simulink model "GFM_GFL_referenceModel_mss_sfunc"  (R2023b)
settings: Solver=ode23  StartTime=0.1  StopTime=1  MaxStep=SimulationSetup.Solver.MaxStep  RelTol=SimulationSetup.Solver.RelTol
undefined symbols (not defined in the file): freq, H, Ibase, K_damping, Kdroop_V, Ki_CC, ki_P, ki_PLL, ki_Q, Kp_CC, kp_P, kp_PLL, kp_Q, Lconv1, Lg, Lv, msys, Qref, Rconv1, Rg, Rv, Sbase, SimulationSetup, Vpeak, wf_PQ, wg, x0
libraries: eeStairGenerator x1
settings Model: Creator=kauchr  LastModifiedBy=weq968
settings DataIOCC: ExternalInput=[tsig, usig]  LoadInitialState=on  SaveFinalState=on  SaveOperatingPoint=on  SaveState=on

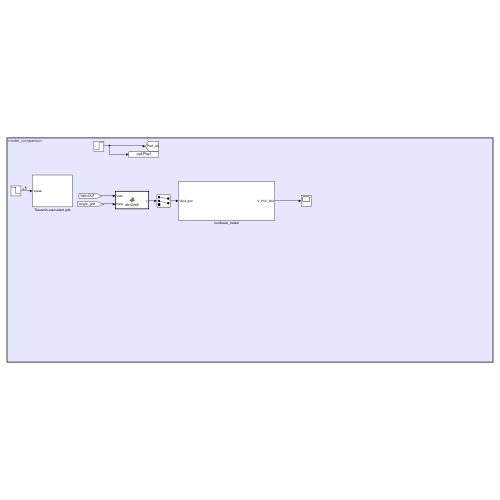
[thumbnail: Simulink's stored preview of the top-level diagram]
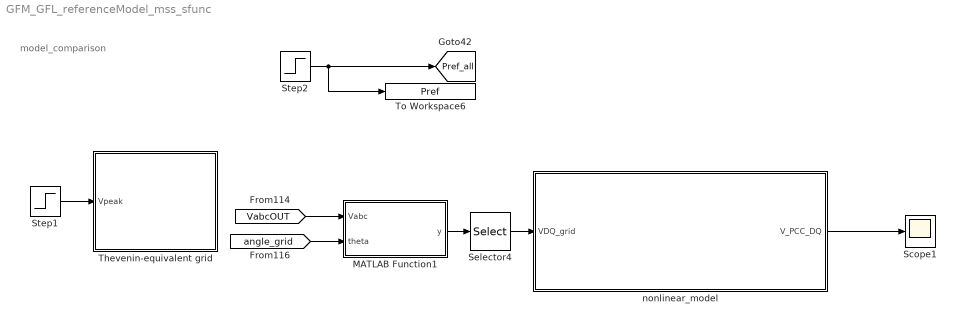
== system GFM_GFL_referenceModel_mss_sfunc ==
  note: model_comparison
  MATLAB Function1 : MATLAB Function  TreatAsAtomicUnit=on
  Scope1 : Scope
  Selector4 : Selector  InputPortWidth=3  IndexOptions=Index vector (dialog)  Indices=[1 2]  OutputSizes=1
  Step1 : Step  Time=SimulationSetup.grid.voltageAmplitudeStep.Time  Before=SimulationSetup.grid.voltageAmplitudeStep.Values(1)  After=SimulationSetup.grid.voltageAmplitudeStep.Values(2)  SampleTime=0
  Step2 : Step  Time=SimulationSetup.converter1.Pref.Time  Before=SimulationSetup.converter1.Pref.Values(1)  After=SimulationSetup.converter1.Pref.Values(2)  SampleTime=0
  Thevenin-equivalent grid : Subsystem
  To Workspace6 : ToWorkspace  VariableName=Pref  SaveFormat=Timeseries  SampleTime=-1
      settings: Save2DSignal=2-D array (concatenate along first dimension)
  nonlinear_model : Subsystem
  tag scope: Pref_all=global
  wires:
  nonlinear_model/1(V_PCC_DQ) -> Scope1/1
  Selector4/1 -> nonlinear_model/1(VDQ_grid)
  [VabcOUT] -> MATLAB Function1/1(Vabc)
  MATLAB Function1/1(y) -> Selector4/1
  [angle_grid] -> MATLAB Function1/2(theta)
  Step1/1 -> Thevenin-equivalent grid/1(Vpeak)
  Step2/1 -> To Workspace6/1, [Pref_all]

== system GFM_GFL_referenceModel_mss_sfunc/Thevenin-equivalent grid ==
  Vpeak : Inport
  Grid : Subsystem
  Mux : Mux  Inputs=3
  tag scope: VabcOUT=global, angle_grid=global
  wires:
  Grid/4(thetareal) -> [angle_grid]
  Grid/2(vzb) -> Mux/2
  Grid/3(vzc) -> Mux/3
  Mux/1 -> [VabcOUT]
  Grid/1(vza) -> Mux/1
  Vpeak/1 -> Grid/1(Vpeak)

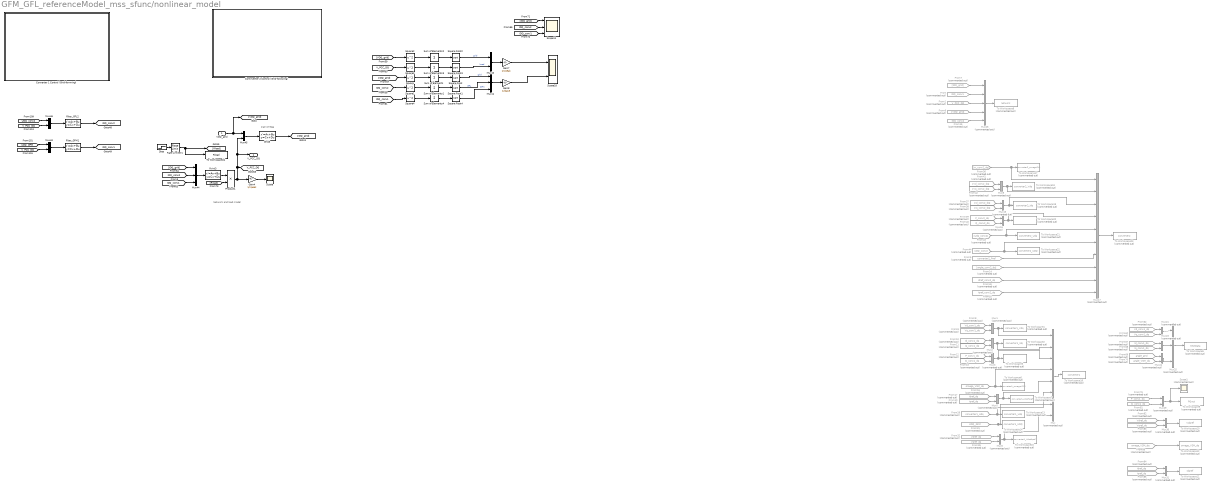
== system GFM_GFL_referenceModel_mss_sfunc/nonlinear_model ==
  note: Network and load model
  note: sign omega
  VDQ_grid : Inport
  Comnverter 2 Control (Grid-following) : Subsystem
  Converter 1 Control (Grid-forrming) : Subsystem
  From : From  Commented=on  GotoTag=IDQ_conv1  TagVisibility=global
  From1 : From  Commented=on  GotoTag=V_PCC_DQ  TagVisibility=global
  From10 : From  Commented=on  GotoTag=Id_conv1_dq  TagVisibility=global
  From11 : From  Commented=on  GotoTag=Iq_conv1_dq  TagVisibility=global
  From12 : From  Commented=on  GotoTag=P_conv1_dq  TagVisibility=global
  From13 : From  Commented=on  GotoTag=Q_conv1_dq  TagVisibility=global
  From14 : From  Commented=on  GotoTag=angle_conv2_dq  TagVisibility=global
  From15 : From  Commented=on  GotoTag=IDQ_conv2  TagVisibility=global
  From16 : From  Commented=on  GotoTag=omega_VSM_dq  TagVisibility=global
  From17 : From  Commented=on  GotoTag=Idref_dq  TagVisibility=global
  From18 : From  Commented=on  GotoTag=Iqref_dq  TagVisibility=global
  From26 : From  Commented=on  GotoTag=converter1_Udq  TagVisibility=global
  From31 : From  Commented=on  GotoTag=UDQ_GFM  TagVisibility=global
  From32 : From  Commented=on  GotoTag=Vdref_dq  TagVisibility=global
  From35 : From  Commented=on  GotoTag=Vqref_dq  TagVisibility=global
  From36 : From  Commented=on  GotoTag=w_conv2_dq  TagVisibility=global
  From37 : From  Commented=on  GotoTag=Id_conv2_dq  TagVisibility=global
  From38 : From  Commented=on  GotoTag=Iq_conv2_dq  TagVisibility=global
  From39 : From  Commented=on  GotoTag=P_conv2_dq  TagVisibility=global
  From40 : From  Commented=on  GotoTag=Q_conv2_dq  TagVisibility=global
  From41 : From  Commented=on  GotoTag=Vd_conv2_dq
  From42 : From  Commented=on  GotoTag=Vq_conv2_dq
  From43 : From  Commented=on  GotoTag=Udq_conv2  TagVisibility=global
  From44 : From  Commented=on  GotoTag=UDQ_conv2  TagVisibility=global
  From45 : From  Commented=on  GotoTag=Idref_conv2_dq  TagVisibility=global
  From5 : From  Commented=on  GotoTag=converter2_Pref  TagVisibility=global
  From55 : From  Commented=on  GotoTag=Iqref_conv2_dq  TagVisibility=global
  From6 : From  Commented=on  GotoTag=VDQ_grid
  From62 : From  Commented=on  GotoTag=Vd_conv1_dq  TagVisibility=global
  From63 : From  Commented=on  GotoTag=Vq_conv1_dq  TagVisibility=global
  From67 : From  Commented=on  GotoTag=Id_conv1_dq  TagVisibility=global
  From68 : From  Commented=on  GotoTag=Iq_conv1_dq  TagVisibility=global
  From69 : From  Commented=on  GotoTag=angle_grid  TagVisibility=global
  From7 : From  Commented=on  GotoTag=IDQ_grid
  From70 : From  Commented=on  GotoTag=angle_VSM_dq  TagVisibility=global
  From76 : From  Commented=on  GotoTag=P_conv1_dq  TagVisibility=global
  From8 : From  Commented=on  GotoTag=Vd_conv1_dq  TagVisibility=global
  From81 : From  Commented=on  GotoTag=Q_conv1_dq  TagVisibility=global
  From82 : From  Commented=on  GotoTag=Vdref_dq  TagVisibility=global
  From83 : From  Commented=on  GotoTag=Vqref_dq  TagVisibility=global
  From84 : From  Commented=on  GotoTag=Idref_dq  TagVisibility=global
  From85 : From  Commented=on  GotoTag=Iqref_dq  TagVisibility=global
  From88 : From  Commented=on  GotoTag=omega_VSM_dq  TagVisibility=global
  From9 : From  Commented=on  GotoTag=Vq_conv1_dq  TagVisibility=global
  Gain4 : Gain  Gain=1/Vpeak
  Gain7 : Gain  Gain=1/Vpeak
  Gain8 : Gain  Gain=1/Ibase
  Grid3 : StateSpace  A=[-Rg/Lg wg; -wg -Rg/Lg]  B=1/Lg*[eye(2),-eye(2)]  C=eye(2)  D=zeros(2,4)  InitialCondition=0  ContinuousStateAttributes='grid_IDQ'
  Mux : Mux  Commented=on  Inputs=[2 2 2 1 2 2 2 2]
  Mux{1..3,5..6,9,15..16,21,23..24,29..31} (14 alike) : Mux  Commented=on  Inputs=2
  Mux10 : Mux  Inputs=2
  Mux11 : Mux  Inputs=3
  Mux17 : Mux  Commented=on  Inputs=[1 2 2 2 2 2 1 1 1 1]
  Mux25 : Mux  Commented=on  Inputs=3
  Mux26 : Mux  Commented=on  Inputs=5
  Mux43 : Mux  Inputs=[2 2]
  Mux44 : Mux  Inputs=[2 2 2]
  Mux45 : Mux  Inputs=[2 2]
  Mux46 : Mux  Inputs=[2 2]
  Product1 : Product
  Rate Limiter1 : RateLimiter  RisingSlewLimit=1000000  FallingSlewLimit=-1000000  SampleTimeMode=inherited
  Rvirt3 : StateSpace  A=[]  B=[]  C=[]  D=[eye(2),eye(2),eye(2)]  InitialCondition=0  ContinuousStateAttributes='VDQ_PCC'
  Scope : Scope
  Scope1 : Scope  Commented=on
  Scope11 : Scope  NumInputPorts=3
  Scope18 : Scope  NumInputPorts=2
  Square{,1..4} (5 alike) : Math  Operator=square
  Square Root{,1..4} (5 alike) : Sqrt
  Step : Step  Time=SimulationSetup.Load.Step.Time  Before=SimulationSetup.Load.Base  After=SimulationSetup.Load.Step.Value  SampleTime=0
  Sum of Elements{,1..4} (5 alike) : Sum  Inputs=+
  To Workspace1 : ToWorkspace  Commented=on  VariableName=converter1_Vdq  SaveFormat=Structure With Time  SampleTime=-1
  To Workspace10 : ToWorkspace  Commented=on  VariableName=Vdqref  SaveFormat=Timeseries  SampleTime=-1
      settings: Save2DSignal=2-D array (concatenate along first dimension)
  To Workspace11 : ToWorkspace  Commented=on  VariableName=Idqref  SaveFormat=Timeseries  SampleTime=-1
      settings: Save2DSignal=2-D array (concatenate along first dimension)
  To Workspace12 : ToWorkspace  Commented=on  VariableName=omega_VSM_dq  SaveFormat=Timeseries  SampleTime=-1
      settings: Save2DSignal=2-D array (concatenate along first dimension)
  To Workspace13 : ToWorkspace  Commented=on  VariableName=converter1_Udq  SaveFormat=Timeseries  SampleTime=-1
      settings: Save2DSignal=2-D array (concatenate along first dimension)
  To Workspace14 : ToWorkspace  Commented=on  VariableName=converter1_UDQ  SaveFormat=Timeseries  SampleTime=-1
      settings: Save2DSignal=2-D array (concatenate along first dimension)
  To Workspace15 : ToWorkspace  Commented=on  VariableName=converter1_Vdrefqref  SaveFormat=Timeseries  SampleTime=-1
      settings: Save2DSignal=2-D array (concatenate along first dimension)
  To Workspace16 : ToWorkspace  Commented=on  VariableName=converter1  SaveFormat=Structure With Time  SampleTime=-1
  To Workspace17 : ToWorkspace  Commented=on  VariableName=converter2_omegaPLL  SaveFormat=Timeseries  SampleTime=-1
      settings: Save2DSignal=2-D array (concatenate along first dimension)
  To Workspace18 : ToWorkspace  Commented=on  VariableName=converter2_Vdq  SaveFormat=Structure With Time  SampleTime=-1
  To Workspace19 : ToWorkspace  Commented=on  VariableName=converter2_Idq  SaveFormat=Structure With Time  SampleTime=-1
  To Workspace2 : ToWorkspace  Commented=on  VariableName=converter1_Idq  SaveFormat=Structure With Time  SampleTime=-1
  To Workspace20 : ToWorkspace  Commented=on  VariableName=converter2_PmeasQmeas  SaveFormat=Structure With Time  SampleTime=-1
  To Workspace21 : ToWorkspace  Commented=on  VariableName=converter2_Udq  SaveFormat=Timeseries  SampleTime=-1
      settings: Save2DSignal=2-D array (concatenate along first dimension)
  To Workspace22 : ToWorkspace  Commented=on  VariableName=converter2_UDQ  SaveFormat=Timeseries  SampleTime=-1
      settings: Save2DSignal=2-D array (concatenate along first dimension)
  To Workspace23 : ToWorkspace  Commented=on  VariableName=converter2  SaveFormat=Structure  SampleTime=-1
      settings: Save2DSignal=2-D array (concatenate along first dimension)
  To Workspace24 : ToWorkspace  VariableName=Rload  SaveFormat=Timeseries  SampleTime=-1
      settings: Save2DSignal=2-D array (concatenate along first dimension)
  To Workspace3 : ToWorkspace  Commented=on  VariableName=converter1_PmeasQmeas  SaveFormat=Structure With Time  SampleTime=-1
  To Workspace5 : ToWorkspace  Commented=on  VariableName=testData  SaveFormat=Structure With Time  SampleTime=-1
  To Workspace6 : ToWorkspace  Commented=on  VariableName=converter1_omegaVSM  SaveFormat=Timeseries  SampleTime=-1
      settings: Save2DSignal=2-D array (concatenate along first dimension)
  To Workspace7 : ToWorkspace  Commented=on  VariableName=converter1_IdrefIqref  SaveFormat=Timeseries  SampleTime=-1
      settings: Save2DSignal=2-D array (concatenate along first dimension)
  To Workspace8 : ToWorkspace  Commented=on  VariableName=network  SaveFormat=Timeseries  SampleTime=-1
      settings: Save2DSignal=2-D array (concatenate along first dimension)
  To Workspace9 : ToWorkspace  Commented=on  VariableName=PQout  SaveFormat=Timeseries  SampleTime=-1
      settings: Save2DSignal=2-D array (concatenate along first dimension)
  filter_GFL2 : StateSpace  A=[-Rconv1/Lconv1 wg; -wg -Rconv1/Lconv1]  B=1/Lconv1*[eye(2),-eye(2)]  C=eye(2)  D=zeros(2,4)  InitialCondition=0  ContinuousStateAttributes='converter2_IDQ'
  filter_GFM1 : StateSpace  A=[-Rconv1/Lconv1 wg; -wg -Rconv1/Lconv1]  B=1/Lconv1*[eye(2),-eye(2)]  C=eye(2)  D=zeros(2,4)  InitialCondition=0  ContinuousStateAttributes='converter1_IDQ'
  V_PCC_DQ : Outport
  tag scope: IDQ_conv1=global, IDQ_conv2=global, V_PCC_DQ=global
  wires:
  Mux29/1 -> Scope1/1, To Workspace9/1
  Mux30/1 -> To Workspace10/1
  Mux31/1 -> To Workspace11/1
  From81/1 -> Mux29/2
  From85/1 -> Mux31/2
  From82/1 -> Mux30/1
  From88/1 -> To Workspace12/1
  From84/1 -> Mux31/1
  From83/1 -> Mux30/2
  From76/1 -> Mux29/1
  From36/1 -> Mux17/1, To Workspace17/1
  From41/1 -> Mux9/1
  Mux9/1 -> Mux17/2, To Workspace18/1
  Mux15/1 -> Mux17/3, To Workspace19/1
  From39/1 -> Mux16/1
  From42/1 -> Mux9/2
  Mux16/1 -> Mux17/4, To Workspace20/1
  From40/1 -> Mux16/2
  From38/1 -> Mux15/2
  From37/1 -> Mux15/1
  From43/1 -> Mux17/5, To Workspace21/1
  From44/1 -> Mux17/6, To Workspace22/1
  Mux17/1 -> To Workspace23/1
  From5/1 -> Mux17/7
  From14/1 -> Mux17/8
  From45/1 -> Mux17/9
  From55/1 -> Mux17/10
  Step/1 -> Rate Limiter1/1
  Gain4/1 -> Scope/1
  filter_GFL2/1 -> [IDQ_conv2]
  [UDQ_conv2] -> Mux46/1
  Mux45/1 -> Grid3/1
  Rvirt3/1 -> Product1/1
  [V_PCC_DQ] -> Mux43/2
  VDQ_grid/1 -> Mux45/1, [VDQ_grid]
  Rate Limiter1/1 -> To Workspace24/1, [Rload]
  Mux43/1 -> filter_GFM1/1
  Grid3/1 -> [IDQ_grid]
  Mux46/1 -> filter_GFL2/1
  [IDQ_conv1] -> Mux44/3
  Product1/1 -> Gain4/1, Mux45/2, V_PCC_DQ/1, [V_PCC_DQ]
  Mux44/1 -> Rvirt3/1
  [UDQ_GFM] -> Mux43/1
  [V_PCC_DQ] -> Mux46/2
  [IDQ_conv2] -> Mux44/2
  [IDQ_grid] -> Mux44/1
  filter_GFM1/1 -> [IDQ_conv1]
  [Rload] -> Product1/2
  Mux5/1 -> Mux/5, To Workspace7/1
  From18/1 -> Mux5/2
  From11/1 -> Mux2/2
  Mux2/1 -> Mux/2, To Workspace2/1
  From13/1 -> Mux3/2
  Mux1/1 -> Mux/1, To Workspace1/1
  Mux3/1 -> Mux/3, To Workspace3/1
  From32/1 -> Mux6/1
  From12/1 -> Mux3/1
  From26/1 -> Mux/6, To Workspace13/1
  Mux6/1 -> Mux/8, To Workspace15/1
  From17/1 -> Mux5/1
  From16/1 -> Mux/4, To Workspace6/1
  From8/1 -> Mux1/1
  From35/1 -> Mux6/2
  From10/1 -> Mux2/1
  Mux/1 -> To Workspace16/1
  From9/1 -> Mux1/2
  From31/1 -> Mux/7, To Workspace14/1
  From62/1 -> Mux21/1
  From70/1 -> Mux24/2
  From68/1 -> Mux23/2
  Mux24/1 -> Mux25/3
  From69/1 -> Mux24/1
  From67/1 -> Mux23/1
  Mux21/1 -> Mux25/1
  Mux23/1 -> Mux25/2
  Mux25/1 -> To Workspace5/1
  From63/1 -> Mux21/2
  From15/1 -> Mux26/5
  Mux26/1 -> To Workspace8/1
  From1/1 -> Mux26/3
  From/1 -> Mux26/2
  From6/1 -> Mux26/4
  From7/1 -> Mux26/1
  [IDQ_grid] -> Scope11/1
  [IDQ_conv1] -> Scope11/3
  [IDQ_conv2] -> Scope11/2
  [IDQ_grid] -> Square/1
  Gain7/1 -> Scope18/1
  [V_PCC_DQ] -> Square3/1
  Mux11/1 -> Gain8/1
  [IDQ_conv1] -> Square4/1
  Sum of Elements1/1 -> Square Root1/1
  Square Root4/1 -> Mux11/3  "GFM"
  Square Root2/1 -> Mux10/1  "grid"
  [VDQ_grid] -> Square2/1
  Square2/1 -> Sum of Elements2/1
  Square/1 -> Sum of Elements/1
  Square Root1/1 -> Mux11/2  "GFL"
  Square1/1 -> Sum of Elements1/1
  Square Root3/1 -> Mux10/2  "load"
  Sum of Elements/1 -> Square Root/1
  Gain8/1 -> Scope18/2
  Mux10/1 -> Gain7/1
  [IDQ_conv2] -> Square1/1
  Sum of Elements3/1 -> Square Root3/1
  Square Root/1 -> Mux11/1  "grid"
  Sum of Elements2/1 -> Square Root2/1
  Sum of Elements4/1 -> Square Root4/1
  Square3/1 -> Sum of Elements3/1
  Square4/1 -> Sum of Elements4/1

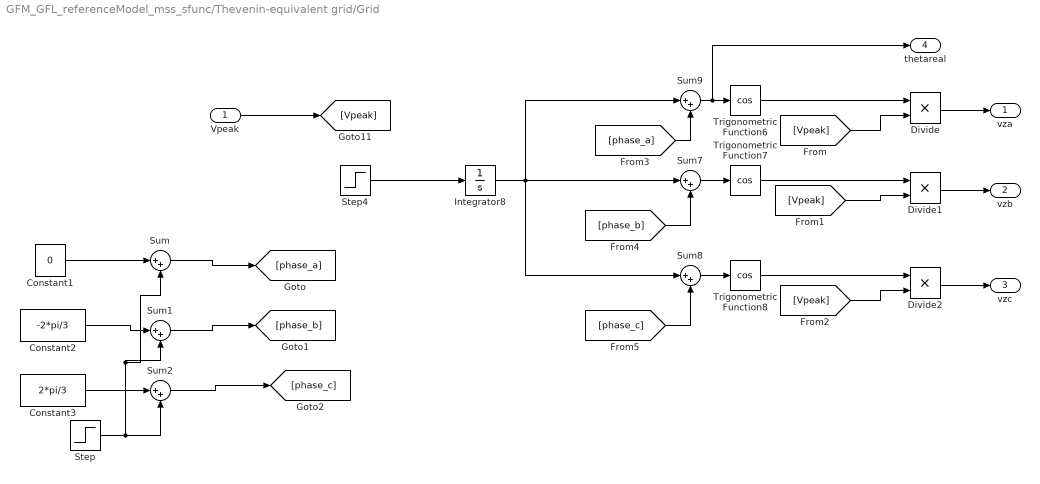
== system GFM_GFL_referenceModel_mss_sfunc/Thevenin-equivalent grid/Grid ==
  Vpeak : Inport
  Constant1 : Constant  Value=0
  Constant2 : Constant  Value=-2*pi/3
  Constant3 : Constant  Value=2*pi/3
  Divide : Product  Inputs=**
  Divide1 : Product  Inputs=**
  Divide2 : Product  Inputs=**
  Integrator8 : Integrator  ContinuousStateAttributes='grid_thetaGRID'
  Step : Step  Time=SimulationSetup.grid.PhaseStep.Time  Before=SimulationSetup.grid.PhaseStep.Values(1)  After=SimulationSetup.grid.PhaseStep.Values(2)  SampleTime=0
  Step4 : Step  Time=SimulationSetup.grid.FrequencyStep.Time  Before=SimulationSetup.grid.FrequencyStep.Values(1)  After=SimulationSetup.grid.FrequencyStep.Values(2)  SampleTime=0
  Sum{,1..2,7..9} (6 alike) : Sum  Inputs=|++
  Trigonometric Function6 : Trigonometry  Operator=cos
  Trigonometric Function7 : Trigonometry  Operator=cos
  Trigonometric Function8 : Trigonometry  Operator=cos
  vza : Outport
  vzb : Outport  Port=2
  vzc : Outport  Port=3
  thetareal : Outport  Port=4
  wires:
  Sum9/1 -> thetareal/1, Trigonometric Function6/1
  [phase_c] -> Sum8/2
  Integrator8/1 -> Sum8/1, Sum9/1, Sum7/1
  [phase_b] -> Sum7/2
  Sum7/1 -> Trigonometric Function7/1
  [phase_a] -> Sum9/2
  Sum8/1 -> Trigonometric Function8/1
  Trigonometric Function6/1 -> Divide/1
  Trigonometric Function7/1 -> Divide1/1
  Trigonometric Function8/1 -> Divide2/1
  Divide/1 -> vza/1
  Divide1/1 -> vzb/1
  Divide2/1 -> vzc/1
  [Vpeak] -> Divide/2
  [Vpeak] -> Divide1/2
  [Vpeak] -> Divide2/2
  Sum1/1 -> [phase_b]
  Sum/1 -> [phase_a]
  Constant1/1 -> Sum/1
  Constant2/1 -> Sum1/1
  Constant3/1 -> Sum2/1
  Sum2/1 -> [phase_c]
  Step/1 -> Sum/2, Sum1/2, Sum2/2
  Step4/1 -> Integrator8/1
  Vpeak/1 -> [Vpeak]

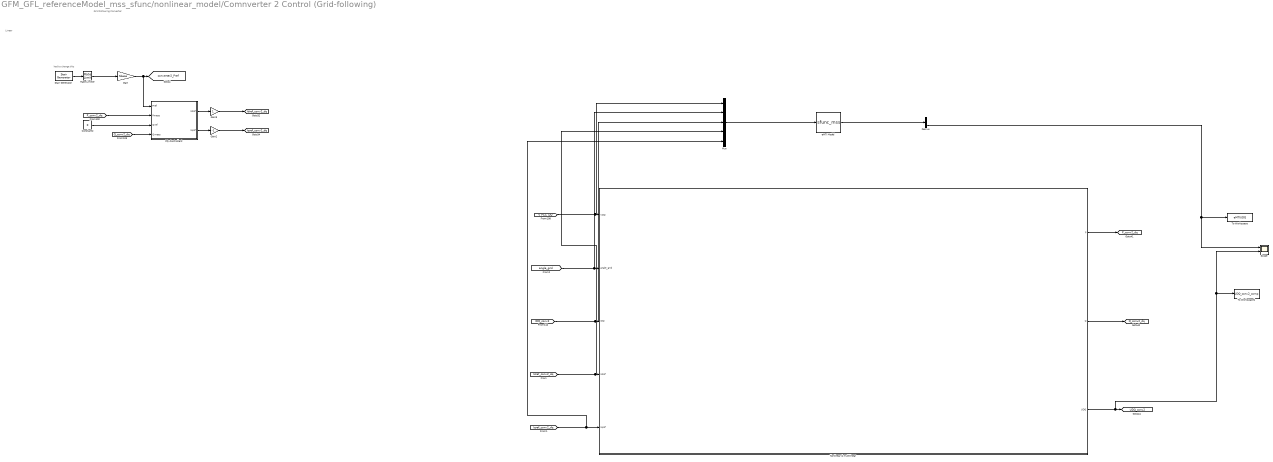
== system GFM_GFL_referenceModel_mss_sfunc/nonlinear_model/Comnverter 2 Control (Grid-following) ==
  note: Linear
  note: Grid Following Converter
  note: had to change this
  Constant2 : Constant  Value=0
  Demux : Demux  Outputs=[1 1 2]
  Gain : Gain  Gain=Sbase
  Gain2 : Gain  Gain=-1
  Gain3 : Gain
  Mux : Mux  Inputs=[2 1 2 1 1]
  Nonlinear & multilinear : Subsystem
  PQ-Controller2 : Subsystem
  Rate Limiter : RateLimiter  RisingSlewLimit=100  FallingSlewLimit=-100  SampleTimeMode=inherited
  Scope : Scope  NumInputPorts=2
  Stair Generator : eeStairGenerator/Stair Generator  LabelModeActiveChoice=Continuous  TimeInput=SimulationSetup.converter2.Pref.Time  AmplitudeInput=SimulationSetup.converter2.Pref.Values  SampleTime=0  RepeatPattern=off  OutDataTypeStr=double
      settings: LibrarySourceBlock=ee_sl_lib/General Control/Stair Generator
  To Workspace : ToWorkspace  VariableName=eMTIUDQ  SaveFormat=Timeseries  SampleTime=-1
  To Workspace1 : ToWorkspace  VariableName=UDQ_conv2_comp  SaveFormat=Timeseries  SampleTime=-1
  eMTI Model : M-S-Function  FunctionName=sfunc_mss  Parameters=msys,x0  mask{msys=msys, x0=x0}
      mask prompts: msys "eMTI model"; x0 "Initial state"
      mask DialogControl eMTI Prompt: This is an implementation of an explicit multilinear (eMTI) model
      mask Display:
      | text(0.5,0.5,'eMTI',...
      |     horizontalAlignment='cente', ...
      |     verticalAlignment = 'middle')
  tag scope: Idref_conv2_dq=global, Iqref_conv2_dq=global, P_conv2_dq=global, Q_conv2_dq=global, UDQ_conv2=global, converter2_Pref=global
  wires:
  PQ-Controller2/2(Iqref) -> Gain2/1
  Gain2/1 -> [Iqref_conv2_dq]
  Gain/1 -> [converter2_Pref], PQ-Controller2/1(Pref)
  Gain3/1 -> [Idref_conv2_dq]
  [P_conv2_dq] -> PQ-Controller2/2(Pmeas)
  PQ-Controller2/1(Idref) -> Gain3/1
  [Q_conv2_dq] -> PQ-Controller2/4(Qmeas)
  Rate Limiter/1 -> Gain/1
  Constant2/1 -> PQ-Controller2/3(Qref)
  Stair Generator/1 -> Rate Limiter/1
  Nonlinear & multilinear/1(P) -> [P_conv2_dq]
  Nonlinear & multilinear/2(Q) -> [Q_conv2_dq]
  [V_PCC_DQ] -> Mux/1, Nonlinear & multilinear/1(VDQ)
  [angle_grid] -> Mux/2, Nonlinear & multilinear/2(angle_grid)
  [IDQ_conv2] -> Mux/3, Nonlinear & multilinear/3(IDQ)
  [Iqref_conv2_dq] -> Mux/5, Nonlinear & multilinear/5(Iqref)
  Nonlinear & multilinear/3(UDQ) -> To Workspace1/1, Scope/2, [UDQ_conv2]
  [Idref_conv2_dq] -> Mux/4, Nonlinear & multilinear/4(Idref)
  Mux/1 -> eMTI Model/1
  eMTI Model/1 -> Demux/1
  Demux/3 -> Scope/1, To Workspace/1

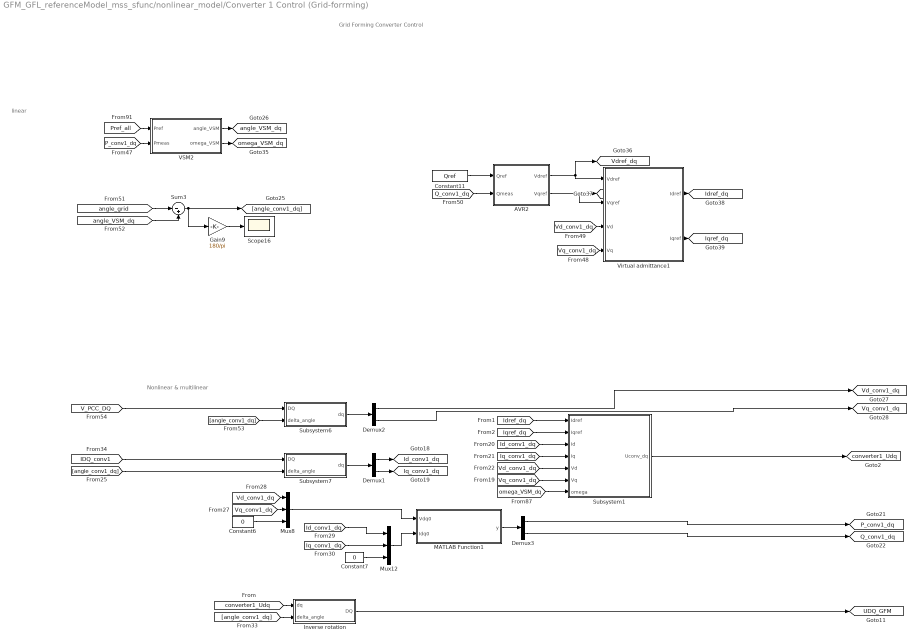
== system GFM_GFL_referenceModel_mss_sfunc/nonlinear_model/Converter 1 Control (Grid-forrming) ==
  note: linear
  note: Nonlinear & multilinear
  note: Grid Forming Converter Control
  AVR2 : Subsystem
  Constant11 : Constant  Value=Qref
  Constant6 : Constant  Value=0
  Constant7 : Constant  Value=0
  Demux1 : Demux  Outputs=2
  Demux2 : Demux  Outputs=2
  Demux3 : Demux  Outputs=2
  Gain9 : Gain  Gain=180/pi
  Inverse rotation : Subsystem
  MATLAB Function1 : MATLAB Function  TreatAsAtomicUnit=on
  Mux12 : Mux  Inputs=3
  Mux8 : Mux  Inputs=3
  Scope16 : Scope
  Subsystem1 : Subsystem
  Subsystem6 : Subsystem
  Subsystem7 : Subsystem
  Sum3 : Sum  Inputs=|-+
  VSM2 : Subsystem
  Virtual admittance1 : Subsystem
  tag scope: Id_conv1_dq=global, Idref_dq=global, Iq_conv1_dq=global, Iqref_dq=global, P_conv1_dq=global, Q_conv1_dq=global, UDQ_GFM=global, Vd_conv1_dq=global, Vdref_dq=global, Vq_conv1_dq=global, Vqref_dq=global, angle_VSM_dq=global, converter1_Udq=global, omega_VSM_dq=global
  wires:
  Virtual admittance1/2(Iqref) -> [Iqref_dq]
  [angle_conv1_dq] -> Inverse rotation/2(delta_angle)
  [Id_conv1_dq] -> Subsystem1/3(Id)
  Mux12/1 -> MATLAB Function1/2(Idq0)
  Sum3/1 -> Gain9/1, [angle_conv1_dq]
  Constant6/1 -> Mux8/3
  Constant11/1 -> AVR2/1(Qref)
  [Id_conv1_dq] -> Mux12/1
  [IDQ_conv1] -> Subsystem7/1(DQ)
  [Vq_conv1_dq] -> Subsystem1/6(Vq)
  [V_PCC_DQ] -> Subsystem6/1(DQ)
  [Vd_conv1_dq] -> Mux8/1
  [angle_conv1_dq] -> Subsystem7/2(delta_angle)
  AVR2/2(Vqref) -> [Vqref_dq], Virtual admittance1/2(Vqref)
  Subsystem1/1(Uconv_dq) -> [converter1_Udq]
  Mux8/1 -> MATLAB Function1/1(Vdq0)
  Gain9/1 -> Scope16/1
  AVR2/1(Vdref) -> [Vdref_dq], Virtual admittance1/1(Vdref)
  Demux1/1 -> [Id_conv1_dq]
  Virtual admittance1/1(Idref) -> [Idref_dq]
  VSM2/1(angle_VSM) -> [angle_VSM_dq]
  [Vd_conv1_dq] -> Virtual admittance1/3(Vd)
  VSM2/2(omega_VSM) -> [omega_VSM_dq]
  [angle_grid] -> Sum3/1
  [Vq_conv1_dq] -> Virtual admittance1/4(Vq)
  Constant7/1 -> Mux12/3
  Subsystem7/1(dq) -> Demux1/1
  [Iq_conv1_dq] -> Subsystem1/4(Iq)
  [P_conv1_dq] -> VSM2/2(Pmeas)
  [angle_conv1_dq] -> Subsystem6/2(delta_angle)
  Demux3/2 -> [Q_conv1_dq]
  [angle_VSM_dq] -> Sum3/2
  Inverse rotation/1(DQ) -> [UDQ_GFM]
  [Q_conv1_dq] -> AVR2/2(Qmeas)
  [Vq_conv1_dq] -> Mux8/2
  Subsystem6/1(dq) -> Demux2/1
  Demux2/2 -> [Vq_conv1_dq]
  Demux2/1 -> [Vd_conv1_dq]
  [Iq_conv1_dq] -> Mux12/2
  Demux1/2 -> [Iq_conv1_dq]
  [omega_VSM_dq] -> Subsystem1/7(omega)
  [Pref_all] -> VSM2/1(Pref)
  [Vd_conv1_dq] -> Subsystem1/5(Vd)
  [converter1_Udq] -> Inverse rotation/1(dq)
  [Idref_dq] -> Subsystem1/1(Idref)
  [Iqref_dq] -> Subsystem1/2(Iqref)
  MATLAB Function1/1(y) -> Demux3/1
  Demux3/1 -> [P_conv1_dq]

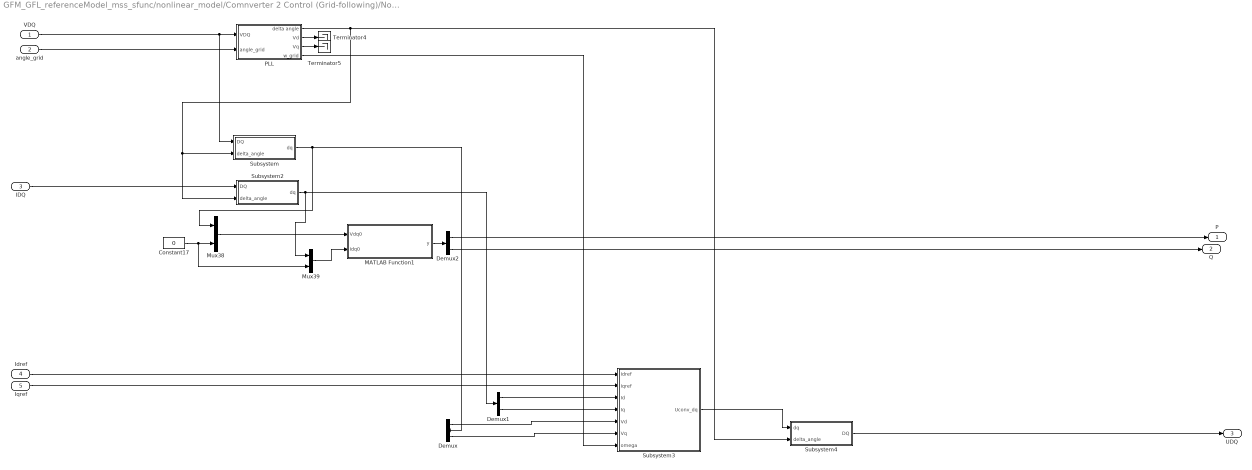
== system GFM_GFL_referenceModel_mss_sfunc/nonlinear_model/Comnverter 2 Control (Grid-following)/Nonlinear & multilinear ==
  VDQ : Inport
  angle_grid : Inport  Port=2
  IDQ : Inport  Port=3
  Idref : Inport  Port=4
  Iqref : Inport  Port=5
  Constant17 : Constant  Value=0
  Demux : Demux  Outputs=2
  Demux1 : Demux  Outputs=2
  Demux2 : Demux  Outputs=2
  MATLAB Function1 : MATLAB Function  TreatAsAtomicUnit=on
  Mux38 : Mux  Inputs=[2 1]
  Mux39 : Mux  Inputs=[2 1]
  PLL : Subsystem
  Subsystem : Subsystem
  Subsystem2 : Subsystem
  Subsystem3 : Subsystem
  Subsystem4 : Subsystem
  Terminator4 : Terminator
  Terminator5 : Terminator
  P : Outport
  Q : Outport  Port=2
  UDQ : Outport  Port=3
  wires:
  Iqref/1 -> Subsystem3/2(Iqref)
  PLL/1(delta angle) -> Subsystem2/2(delta_angle), Subsystem/2(delta_angle), Subsystem4/2(delta_angle)
  Subsystem/1(dq) -> Mux38/1, Demux/1
  Demux2/2 -> Q/1
  Subsystem4/1(DQ) -> UDQ/1
  Constant17/1 -> Mux39/2, Mux38/2
  Demux1/2 -> Subsystem3/4(Iq)
  VDQ/1 -> Subsystem/1(DQ), PLL/1(VDQ)
  Demux/2 -> Subsystem3/6(Vq)
  Subsystem2/1(dq) -> Mux39/1, Demux1/1
  PLL/4(w_grid) -> Subsystem3/7(omega)
  PLL/3(Vq) -> Terminator5/1
  PLL/2(Vd) -> Terminator4/1
  Idref/1 -> Subsystem3/1(Idref)
  Mux38/1 -> MATLAB Function1/1(Vdq0)
  Mux39/1 -> MATLAB Function1/2(Idq0)
  Subsystem3/1(Uconv_dq) -> Subsystem4/1(dq)
  Demux1/1 -> Subsystem3/3(Id)
  Demux/1 -> Subsystem3/5(Vd)
  Demux2/1 -> P/1
  IDQ/1 -> Subsystem2/1(DQ)
  angle_grid/1 -> PLL/2(angle_grid)
  MATLAB Function1/1(y) -> Demux2/1

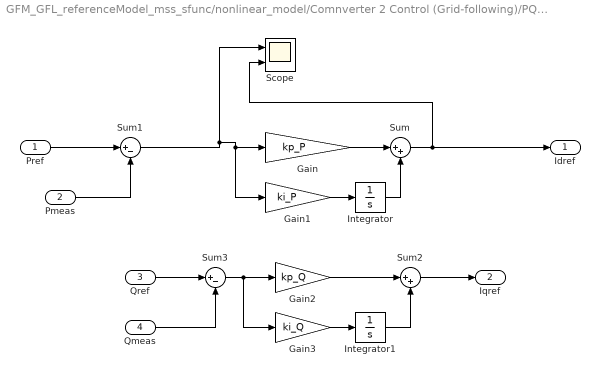
== system GFM_GFL_referenceModel_mss_sfunc/nonlinear_model/Comnverter 2 Control (Grid-following)/PQ-Controller2 ==
  Pref : Inport
  Pmeas : Inport  Port=2
  Qref : Inport  Port=3
  Qmeas : Inport  Port=4
  Gain : Gain  Gain=kp_P
  Gain1 : Gain  Gain=ki_P
  Gain2 : Gain  Gain=kp_Q
  Gain3 : Gain  Gain=ki_Q
  Integrator : Integrator  ContinuousStateAttributes='converter2_xI_Pctrl'
  Integrator1 : Integrator  ContinuousStateAttributes='converter2_xI_Qctrl'
  Scope : Scope  NumInputPorts=2
  Sum : Sum  Inputs=|++
  Sum1 : Sum  Inputs=|+-
  Sum2 : Sum  Inputs=|++
  Sum3 : Sum  Inputs=|+-
  Idref : Outport
  Iqref : Outport  Port=2
  wires:
  Gain1/1 -> Integrator/1
  Integrator/1 -> Sum/2
  Gain/1 -> Sum/1
  Sum/1 -> Idref/1, Scope/2
  Pmeas/1 -> Sum1/2
  Integrator1/1 -> Sum2/2
  Sum2/1 -> Iqref/1
  Sum3/1 -> Gain3/1, Gain2/1
  Gain2/1 -> Sum2/1
  Qmeas/1 -> Sum3/2
  Gain3/1 -> Integrator1/1
  Qref/1 -> Sum3/1
  Sum1/1 -> Scope/1, Gain1/1, Gain/1
  Pref/1 -> Sum1/1

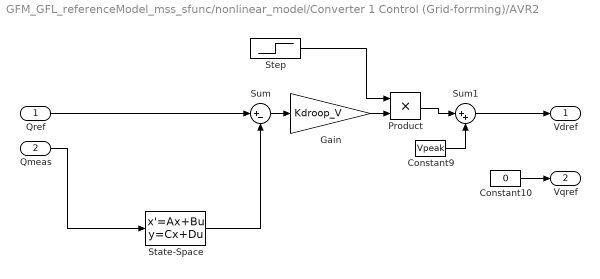
== system GFM_GFL_referenceModel_mss_sfunc/nonlinear_model/Converter 1 Control (Grid-forrming)/AVR2 ==
  Qref : Inport
  Qmeas : Inport  Port=2
  Constant10 : Constant  Value=0
  Constant9 : Constant  Value=Vpeak
  Gain : Gain  Gain=Kdroop_V
  Product : Product
  State-Space : StateSpace  A=-wf_PQ  B=wf_PQ  D=0  InitialCondition=0  ContinuousStateAttributes='converter1_xI_Vdroop'
  Step : Step  Time=SimulationSetup.converter1.VoltageCtrl.ActivationTime  SampleTime=0
  Sum : Sum  Inputs=|+-
  Sum1 : Sum  Inputs=|++
  Vdref : Outport
  Vqref : Outport  Port=2
  wires:
  Qref/1 -> Sum/1
  Constant9/1 -> Sum1/2
  Sum/1 -> Gain/1
  Qmeas/1 -> State-Space/1
  Product/1 -> Sum1/1
  Step/1 -> Product/1
  Gain/1 -> Product/2
  State-Space/1 -> Sum/2
  Sum1/1 -> Vdref/1
  Constant10/1 -> Vqref/1

== system GFM_GFL_referenceModel_mss_sfunc/nonlinear_model/Converter 1 Control (Grid-forrming)/Inverse rotation ==
  dq : Inport
  delta_angle : Inport  Port=2
  Gain : Gain
  Gain1 : Gain  Gain=-1
  Matrix Concatenate : Concatenate  Mode=Multidimensional array  ConcatenateDimension=2
  Mux : Mux  Inputs=2
  Mux1 : Mux  Inputs=2
  Product : Product  Multiplication=Matrix(*)
  Sin : Trigonometry
  Sin1 : Trigonometry  Operator=cos
  DQ : Outport
  wires:
  Matrix Concatenate/1 -> Product/1
  dq/1 -> Product/2
  Product/1 -> DQ/1
  delta_angle/1 -> Sin1/1, Sin/1
  Sin1/1 -> Mux1/2, Mux/1
  Sin/1 -> Gain1/1, Gain/1
  Gain/1 -> Mux/2
  Mux/1 -> Matrix Concatenate/1
  Mux1/1 -> Matrix Concatenate/2
  Gain1/1 -> Mux1/1

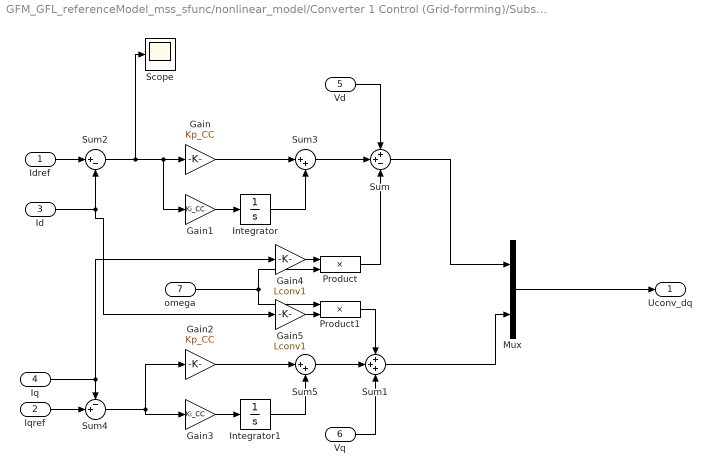
== system GFM_GFL_referenceModel_mss_sfunc/nonlinear_model/Converter 1 Control (Grid-forrming)/Subsystem1 ==
  Idref : Inport
  Iqref : Inport  Port=2
  Id : Inport  Port=3
  Iq : Inport  Port=4
  Vd : Inport  Port=5
  Vq : Inport  Port=6
  omega : Inport  Port=7
  Gain : Gain  Gain=Kp_CC
  Gain1 : Gain  Gain=Ki_CC
  Gain2 : Gain  Gain=Kp_CC
  Gain3 : Gain  Gain=Ki_CC
  Gain4 : Gain  Gain=Lconv1
  Gain5 : Gain  Gain=Lconv1
  Integrator : Integrator  ContinuousStateAttributes='converter1_xId_CC'
  Integrator1 : Integrator  ContinuousStateAttributes='converter1_xIq_CC'
  Mux : Mux  Inputs=2
  Product : Product
  Product1 : Product
  Scope : Scope
  Sum : Sum  Inputs=++-
  Sum1 : Sum  Inputs=+++
  Sum2 : Sum  Inputs=|+-
  Sum3 : Sum  Inputs=|++
  Sum4 : Sum  Inputs=-+|
  Sum5 : Sum  Inputs=|++
  Uconv_dq : Outport
  wires:
  Vd/1 -> Sum/1
  Vq/1 -> Sum1/3
  Sum/1 -> Mux/1
  Sum1/1 -> Mux/2
  Mux/1 -> Uconv_dq/1
  Idref/1 -> Sum2/1
  Id/1 -> Sum2/2, Gain5/1
  Sum2/1 -> Scope/1, Gain1/1, Gain/1
  Gain1/1 -> Integrator/1
  Integrator/1 -> Sum3/2
  Gain/1 -> Sum3/1
  Sum3/1 -> Sum/2
  Iqref/1 -> Sum4/2
  Iq/1 -> Gain4/1, Sum4/1
  Integrator1/1 -> Sum5/2
  Sum5/1 -> Sum1/2
  Gain3/1 -> Integrator1/1
  Gain2/1 -> Sum5/1
  Sum4/1 -> Gain2/1, Gain3/1
  Gain4/1 -> Product/1
  Product/1 -> Sum/3
  omega/1 -> Product/2, Product1/1
  Gain5/1 -> Product1/2
  Product1/1 -> Sum1/1

== system GFM_GFL_referenceModel_mss_sfunc/nonlinear_model/Converter 1 Control (Grid-forrming)/Subsystem6 ==
  DQ : Inport
  delta_angle : Inport  Port=2
  Gain : Gain  Gain=-1
  Matrix Concatenate : Concatenate  Mode=Multidimensional array  ConcatenateDimension=2
  Mux : Mux  Inputs=2
  Mux1 : Mux  Inputs=2
  Product : Product  Multiplication=Matrix(*)
  Sin : Trigonometry
  Sin1 : Trigonometry  Operator=cos
  dq : Outport
  wires:
  Matrix Concatenate/1 -> Product/1
  DQ/1 -> Product/2
  Product/1 -> dq/1
  delta_angle/1 -> Sin1/1, Sin/1
  Sin1/1 -> Mux1/2, Mux/1
  Sin/1 -> Mux1/1, Gain/1
  Gain/1 -> Mux/2
  Mux/1 -> Matrix Concatenate/1
  Mux1/1 -> Matrix Concatenate/2

== system GFM_GFL_referenceModel_mss_sfunc/nonlinear_model/Converter 1 Control (Grid-forrming)/Subsystem7 ==
  DQ : Inport
  delta_angle : Inport  Port=2
  Gain : Gain  Gain=-1
  Matrix Concatenate : Concatenate  Mode=Multidimensional array  ConcatenateDimension=2
  Mux : Mux  Inputs=2
  Mux1 : Mux  Inputs=2
  Product : Product  Multiplication=Matrix(*)
  Sin : Trigonometry
  Sin1 : Trigonometry  Operator=cos
  dq : Outport
  wires:
  Matrix Concatenate/1 -> Product/1
  DQ/1 -> Product/2
  Product/1 -> dq/1
  delta_angle/1 -> Sin1/1, Sin/1
  Sin1/1 -> Mux1/2, Mux/1
  Sin/1 -> Mux1/1, Gain/1
  Gain/1 -> Mux/2
  Mux/1 -> Matrix Concatenate/1
  Mux1/1 -> Matrix Concatenate/2

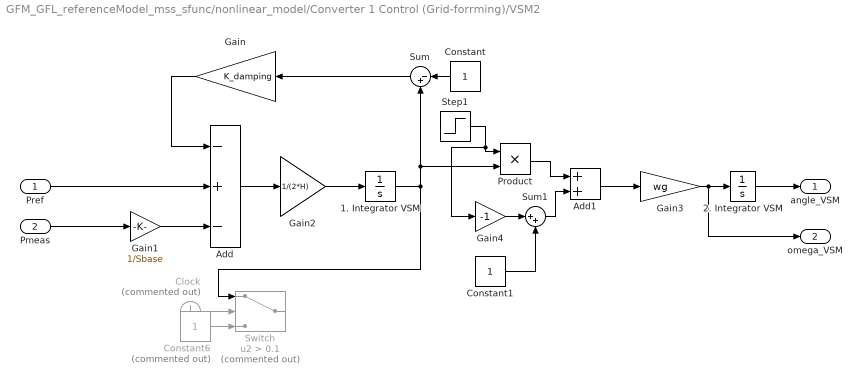
== system GFM_GFL_referenceModel_mss_sfunc/nonlinear_model/Converter 1 Control (Grid-forrming)/VSM2 ==
  Pref : Inport
  Pmeas : Inport  Port=2
  1. Integrator VSM : Integrator  ContinuousStateAttributes='converter1_xI_vsm'
  2. Integrator VSM : Integrator  ContinuousStateAttributes='converter1_thetaVSM'
  Add : Sum  Inputs=-+-
  Add1 : Sum
  Clock : Clock  Commented=on
  Constant : Constant
  Constant1 : Constant
  Constant6 : Constant  Commented=on
  Gain : Gain  Gain=K_damping
  Gain1 : Gain  Gain=1/Sbase
  Gain2 : Gain  Gain=1/(2*H)
  Gain3 : Gain  Gain=wg
  Gain4 : Gain  Gain=-1
  Product : Product
  Step1 : Step  Time=SimulationSetup.converter1.FreqCtrl.ActivationTime  SampleTime=0
  Sum : Sum  Inputs=|-+
  Sum1 : Sum  Inputs=|++
  Switch : Switch  Commented=on  Criteria=u2 > Threshold  Threshold=0.1  SaturateOnIntegerOverflow=off  InputSameDT=off
  angle_VSM : Outport
  omega_VSM : Outport  Port=2
  wires:
  Pmeas/1 -> Gain1/1
  Gain2/1 -> 1. Integrator VSM/1
  Pref/1 -> Add/2
  Gain1/1 -> Add/3
  Add/1 -> Gain2/1
  1. Integrator VSM/1 -> Product/2, Sum/2, Switch/1
  Constant/1 -> Sum/1
  Sum/1 -> Gain/1
  Gain/1 -> Add/1
  Gain3/1 -> omega_VSM/1, 2. Integrator VSM/1
  2. Integrator VSM/1 -> angle_VSM/1
  Clock/1 -> Switch/2
  Constant6/1 -> Switch/3
  Add1/1 -> Gain3/1
  Product/1 -> Add1/1
  Step1/1 -> Gain4/1, Product/1
  Gain4/1 -> Sum1/1
  Sum1/1 -> Add1/2
  Constant1/1 -> Sum1/2

== system GFM_GFL_referenceModel_mss_sfunc/nonlinear_model/Converter 1 Control (Grid-forrming)/Virtual admittance1 ==
  Vdref : Inport
  Vqref : Inport  Port=2
  Vd : Inport  Port=3
  Vq : Inport  Port=4
  Demux : Demux  Outputs=2
  Mux : Mux  Inputs=2
  State-Space : StateSpace  A=[-Rv/Lv, +wg; -wg, -Rv/Lv]  B=[1 0; 0 1]  C=1/Lv*eye(2)  D=zeros(2,2)  InitialCondition=0  ContinuousStateAttributes={'converter1_xId_VA','converter1_xIq_VA'}
  Sum2 : Sum  Inputs=|+-
  Sum4 : Sum  Inputs=-+|
  Idref : Outport
  Iqref : Outport  Port=2
  wires:
  Vdref/1 -> Sum2/1
  Vd/1 -> Sum2/2
  Vqref/1 -> Sum4/2
  Vq/1 -> Sum4/1
  Sum2/1 -> Mux/1
  Sum4/1 -> Mux/2
  Mux/1 -> State-Space/1
  State-Space/1 -> Demux/1
  Demux/1 -> Idref/1
  Demux/2 -> Iqref/1

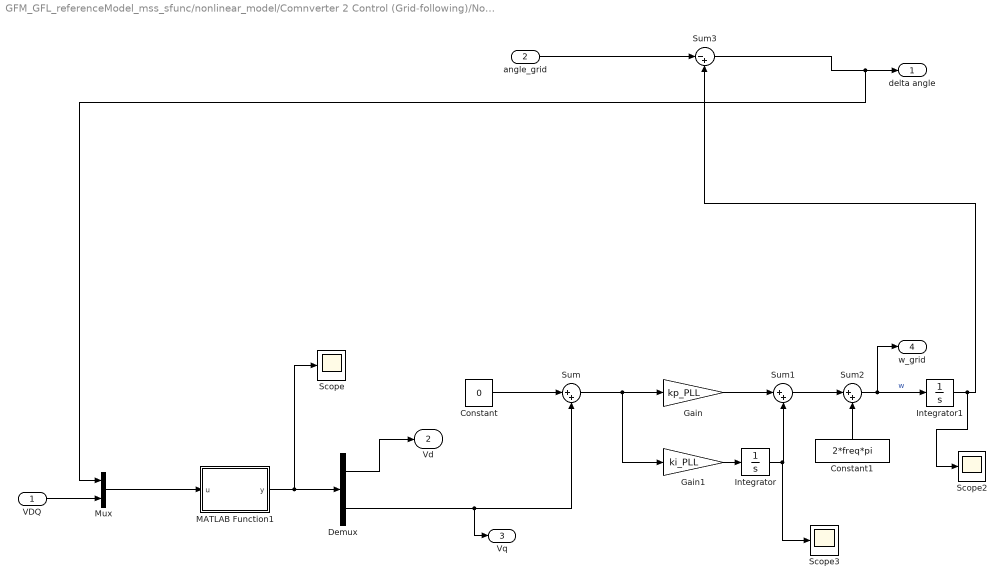
== system GFM_GFL_referenceModel_mss_sfunc/nonlinear_model/Comnverter 2 Control (Grid-following)/Nonlinear & multilinear/PLL ==
  VDQ : Inport
  angle_grid : Inport  Port=2
  Constant : Constant  Value=0
  Constant1 : Constant  Value=2*freq*pi
  Demux : Demux  Outputs=2
  Gain : Gain  Gain=kp_PLL
  Gain1 : Gain  Gain=ki_PLL
  Integrator : Integrator  ContinuousStateAttributes='converter2_xI_PLL'
  Integrator1 : Integrator  ContinuousStateAttributes='converter2_thetaPLL'
  MATLAB Function1 : MATLAB Function  TreatAsAtomicUnit=on
  Mux : Mux  Inputs=[1 2]
  Scope : Scope
  Scope2 : Scope
  Scope3 : Scope
  Sum : Sum  Inputs=|++
  Sum1 : Sum  Inputs=|++
  Sum2 : Sum  Inputs=|++
  Sum3 : Sum  Inputs=|-+
  delta angle : Outport
  Vd : Outport  Port=2
  Vq : Outport  Port=3
  w_grid : Outport  Port=4
  wires:
  Sum1/1 -> Sum2/1
  Gain/1 -> Sum1/1
  Integrator/1 -> Scope3/1, Sum1/2
  Gain1/1 -> Integrator/1
  Demux/1 -> Vd/1
  Sum2/1 -> w_grid/1, Integrator1/1  "w"
  Constant/1 -> Sum/1
  Constant1/1 -> Sum2/2
  MATLAB Function1/1(y) -> Scope/1, Demux/1
  VDQ/1 -> Mux/2
  Sum/1 -> Gain1/1, Gain/1
  Mux/1 -> MATLAB Function1/1(u)
  Demux/2 -> Vq/1, Sum/2
  Integrator1/1 -> Scope2/1, Sum3/2
  Sum3/1 -> Mux/1, delta angle/1
  angle_grid/1 -> Sum3/1

== system GFM_GFL_referenceModel_mss_sfunc/nonlinear_model/Comnverter 2 Control (Grid-following)/Nonlinear & multilinear/Subsystem ==
  DQ : Inport
  delta_angle : Inport  Port=2
  Gain : Gain  Gain=-1
  Matrix Concatenate : Concatenate  Mode=Multidimensional array  ConcatenateDimension=2
  Mux : Mux  Inputs=2
  Mux1 : Mux  Inputs=2
  Product : Product  Multiplication=Matrix(*)
  Sin : Trigonometry
  Sin1 : Trigonometry  Operator=cos
  dq : Outport
  wires:
  Matrix Concatenate/1 -> Product/1
  DQ/1 -> Product/2
  Product/1 -> dq/1
  delta_angle/1 -> Sin1/1, Sin/1
  Sin1/1 -> Mux1/2, Mux/1
  Sin/1 -> Mux1/1, Gain/1
  Gain/1 -> Mux/2
  Mux/1 -> Matrix Concatenate/1
  Mux1/1 -> Matrix Concatenate/2

== system GFM_GFL_referenceModel_mss_sfunc/nonlinear_model/Comnverter 2 Control (Grid-following)/Nonlinear & multilinear/Subsystem2 ==
  DQ : Inport
  delta_angle : Inport  Port=2
  Gain : Gain  Gain=-1
  Matrix Concatenate : Concatenate  Mode=Multidimensional array  ConcatenateDimension=2
  Mux : Mux  Inputs=2
  Mux1 : Mux  Inputs=2
  Product : Product  Multiplication=Matrix(*)
  Sin : Trigonometry
  Sin1 : Trigonometry  Operator=cos
  dq : Outport
  wires:
  Matrix Concatenate/1 -> Product/1
  DQ/1 -> Product/2
  Product/1 -> dq/1
  delta_angle/1 -> Sin1/1, Sin/1
  Sin1/1 -> Mux1/2, Mux/1
  Sin/1 -> Mux1/1, Gain/1
  Gain/1 -> Mux/2
  Mux/1 -> Matrix Concatenate/1
  Mux1/1 -> Matrix Concatenate/2

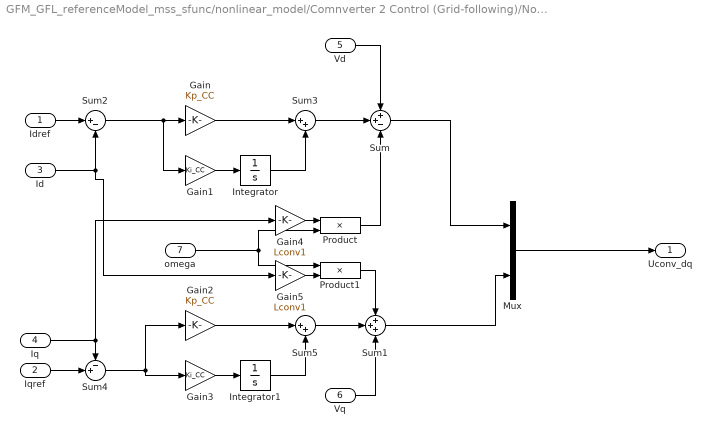
== system GFM_GFL_referenceModel_mss_sfunc/nonlinear_model/Comnverter 2 Control (Grid-following)/Nonlinear & multilinear/Subsystem3 ==
  Idref : Inport
  Iqref : Inport  Port=2
  Id : Inport  Port=3
  Iq : Inport  Port=4
  Vd : Inport  Port=5
  Vq : Inport  Port=6
  omega : Inport  Port=7
  Gain : Gain  Gain=Kp_CC
  Gain1 : Gain  Gain=Ki_CC
  Gain2 : Gain  Gain=Kp_CC
  Gain3 : Gain  Gain=Ki_CC
  Gain4 : Gain  Gain=Lconv1
  Gain5 : Gain  Gain=Lconv1
  Integrator : Integrator  ContinuousStateAttributes='converter2_xId_CC'
  Integrator1 : Integrator  ContinuousStateAttributes='converter2_xIq_CC'
  Mux : Mux  Inputs=2
  Product : Product
  Product1 : Product
  Sum : Sum  Inputs=++-
  Sum1 : Sum  Inputs=+++
  Sum2 : Sum  Inputs=|+-
  Sum3 : Sum  Inputs=|++
  Sum4 : Sum  Inputs=-+|
  Sum5 : Sum  Inputs=|++
  Uconv_dq : Outport
  wires:
  Vd/1 -> Sum/1
  Vq/1 -> Sum1/3
  Sum/1 -> Mux/1
  Sum1/1 -> Mux/2
  Mux/1 -> Uconv_dq/1
  Idref/1 -> Sum2/1
  Id/1 -> Sum2/2, Gain5/1
  Sum2/1 -> Gain1/1, Gain/1
  Gain1/1 -> Integrator/1
  Integrator/1 -> Sum3/2
  Gain/1 -> Sum3/1
  Sum3/1 -> Sum/2
  Iqref/1 -> Sum4/2
  Iq/1 -> Gain4/1, Sum4/1
  Integrator1/1 -> Sum5/2
  Sum5/1 -> Sum1/2
  Gain3/1 -> Integrator1/1
  Gain2/1 -> Sum5/1
  Sum4/1 -> Gain2/1, Gain3/1
  Gain4/1 -> Product/1
  Product/1 -> Sum/3
  omega/1 -> Product/2, Product1/1
  Gain5/1 -> Product1/2
  Product1/1 -> Sum1/1

== system GFM_GFL_referenceModel_mss_sfunc/nonlinear_model/Comnverter 2 Control (Grid-following)/Nonlinear & multilinear/Subsystem4 ==
  dq : Inport
  delta_angle : Inport  Port=2
  Gain : Gain
  Gain1 : Gain  Gain=-1
  Matrix Concatenate : Concatenate  Mode=Multidimensional array  ConcatenateDimension=2
  Mux : Mux  Inputs=2
  Mux1 : Mux  Inputs=2
  Product : Product  Multiplication=Matrix(*)
  Sin : Trigonometry
  Sin1 : Trigonometry  Operator=cos
  DQ : Outport
  wires:
  Matrix Concatenate/1 -> Product/1
  dq/1 -> Product/2
  Product/1 -> DQ/1
  delta_angle/1 -> Sin1/1, Sin/1
  Sin1/1 -> Mux1/2, Mux/1
  Sin/1 -> Gain1/1, Gain/1
  Gain/1 -> Mux/2
  Mux/1 -> Matrix Concatenate/1
  Mux1/1 -> Matrix Concatenate/2
  Gain1/1 -> Mux1/1

== matlab function GFM_GFL_referenceModel_mss_sfunc/nonlinear_model/Converter 1 Control (Grid-forrming)/MATLAB Function1 ==
  data: Vdq0 input; y output; Idq0 input
function y = PQcalculation(Vdq0,Idq0)
 % alignment with d-axis
y =3/2*([Vdq0(1)*Idq0(1)+Vdq0(2)*Idq0(2)+2*Vdq0(3)*Idq0(3);Vdq0(2)*Idq0(1)-Vdq0(1)*Idq0(2);]);

== matlab function GFM_GFL_referenceModel_mss_sfunc/nonlinear_model/Comnverter 2 Control (Grid-following)/Nonlinear & multilinear/MATLAB Function1 ==
  data: Vdq0 input; y output; Idq0 input
function y = PQcalculation(Vdq0,Idq0)
 % alignment with d-axis
y =3/2*([Vdq0(1)*Idq0(1)+Vdq0(2)*Idq0(2)+2*Vdq0(3)*Idq0(3);Vdq0(2)*Idq0(1)-Vdq0(1)*Idq0(2);]);

== matlab function GFM_GFL_referenceModel_mss_sfunc/nonlinear_model/Comnverter 2 Control (Grid-following)/Nonlinear & multilinear/PLL/MATLAB Function1 ==
  data: u input; y output
function y = DQ2dq(u)
 
y =([cos(u(1)), sin(u(1)); -sin(u(1)), cos(u(1))])*[u(2);u(3)];

== matlab function GFM_GFL_referenceModel_mss_sfunc/MATLAB Function1 ==
  data: Vabc input; y output; theta input
function y = abc2dq0(Vabc,theta)
 % alignment with d-axis
y =2/3*([cos(theta), cos(theta-2*pi/3),cos(theta+2*pi/3); -sin(theta), -sin(theta-2*pi/3), -sin(theta+2*pi/3); sqrt(0.5),sqrt(0.5),sqrt(0.5) ])*[Vabc(1);Vabc(2);Vabc(3)];
